simulink model "FullObserver"  (R2017a)
settings: Solver=VariableStepAuto  StartTime=0.0  StopTime=010.0  RelTol=1e-3
undefined symbols (not defined in the file): A, B, C, c, D, F, K, m, n, x0
settings Model: Creator=AMAN  LastModifiedBy=Amit

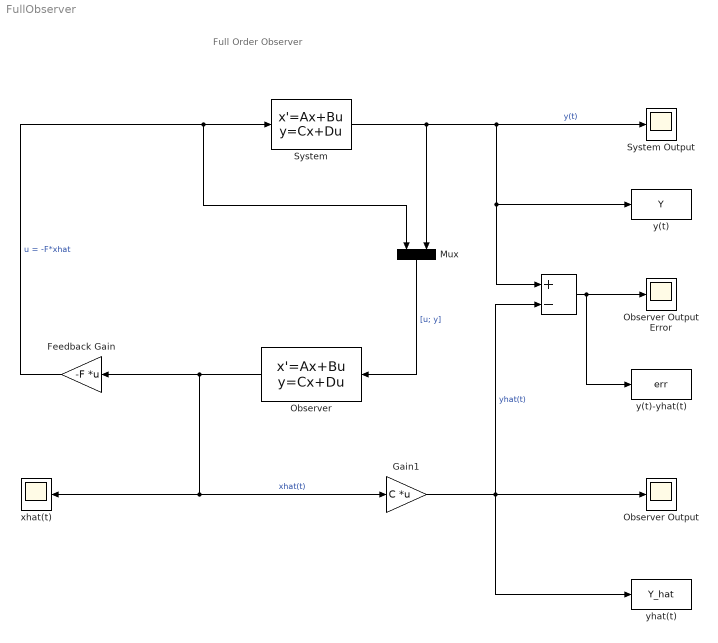
== system FullObserver ==
  note: Full Order Observer
  " " : Sum  Inputs=+-
  Feedback Gain : Gain  Gain=-F  Multiplication=Matrix(K*u)
  Gain1 : Gain  Gain=C  Multiplication=Matrix(K*u)
  Mux : Mux  Inputs=2
  Observer : StateSpace  A=A-K*C  B=[B K]  C=eye(n)  D=zeros(n,m+c)  X0=[0;0;0;0]
  Observer Output : Scope
  Observer Output Error : Scope
  System : StateSpace  A=A  B=B  C=C  D=D  X0=x0
  System Output : Scope
  xhat(t) : Scope
  y(t) : ToWorkspace  VariableName=Y  SaveFormat=Timeseries  SampleTime=-1
  y(t)-yhat(t) : ToWorkspace  VariableName=err  SaveFormat=Timeseries  SampleTime=-1
  yhat(t) : ToWorkspace  VariableName=Y_hat  SaveFormat=Timeseries  SampleTime=-1
  wires:
  Feedback Gain/1 -> System/1, Mux/1  "u = -F*xhat"
  Observer/1 -> Gain1/1, xhat(t)/1, Feedback Gain/1  "xhat(t)"
  Mux/1 -> Observer/1  "[u; y]"
  System/1 -> " "/1, y(t)/1, System Output/1, Mux/2  "y(t)"
  Gain1/1 -> " "/2, yhat(t)/1, Observer Output/1  "yhat(t)"
  " "/1 -> y(t)-yhat(t)/1, Observer Output Error/1
